simulink model "gm_sampleModel1484_2_sub"  (R2023a)
settings: Solver=VariableStepAuto  StartTime=0.0  StopTime=10.0  RelTol=1e-3
libraries: hdlsllib x2, simulink x2
settings Model: Creator=user1  LastModifiedBy=user1
settings OptimizationCC: BlockReduction=off  ConditionallyExecuteInputs=off
settings DebuggingCC: InheritedTsInSrcMsg=none

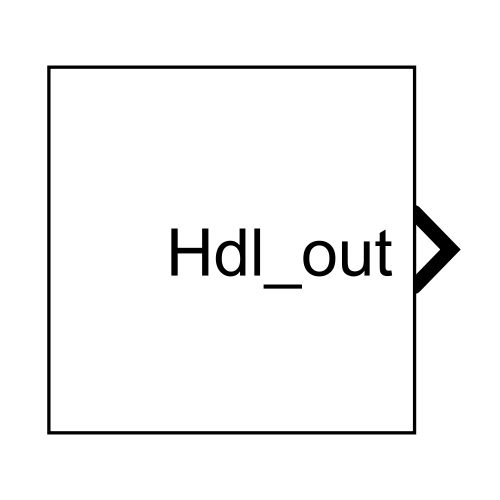
[thumbnail: Simulink's stored preview of the top-level diagram]
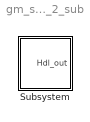
== system gm_sampleModel1484_2_sub ==
  Subsystem : Subsystem

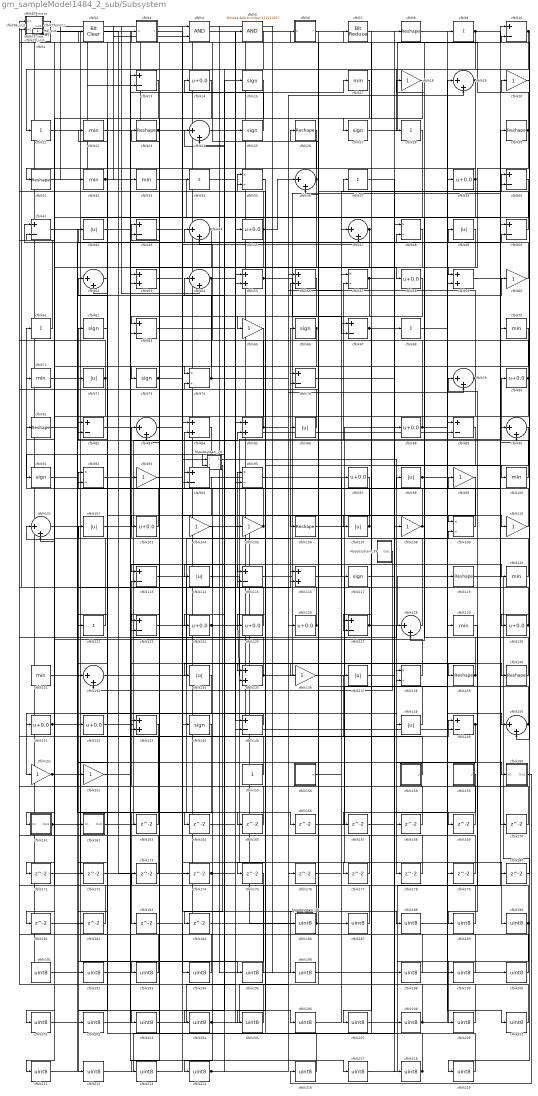
== system gm_sampleModel1484_2_sub/Subsystem ==
  Mysubsystem_20 : Subsystem
  Mysubsystem_38 : Subsystem
  Mysubsystem_39 : Subsystem
  cfblk1 : hdlsllib/Logic and Bit Operations/Bit Concat  numInputs=2
  cfblk{10,13,40..41,43,50,63,67,76,82,89,94,113,115,123,127,145,149} (18 alike) : Sum  Inputs=+-  OutDataTypeStr=uint8
  cfblk{17,22,32..33,70..71,100,120,129,131} (10 alike) : MinMax  OutDataTypeStr=uint8
  cfblk{19,24,36,44,47,52,54,79,83,90,101,128,132,150} (14 alike) : Sum  Inputs=|++  OutDataTypeStr=uint8
  cfblk{42,49,72,86,98,102,107,114,134,137,148} (11 alike) : Abs  OutDataTypeStr=uint8  SaturateOnIntegerOverflow=off
  cfblk{14,39,45,58,80,88,97,103,124..126,130,141..142} (14 alike) : Bias  Bias=0.0  SaturateOnIntegerOverflow=off
  cfblk{18,20,60,65,93,99,104..105,108,110,136,151..152} (13 alike) : Gain  OutDataTypeStr=uint8
  cfblk{8,23,26,30..31,81,106,119,139..140} (10 alike) : Reshape
  cfblk{35,48,57,74,92,95,109,138} (8 alike) : Product  Inputs=*/  OutDataTypeStr=uint8  RndMeth=Zero  SaturateOnIntegerOverflow=on
  cfblk112_inst : Subsystem
  cfblk{53,55..56,59,84..85,116,135,143} (9 alike) : Sum  OutDataTypeStr=uint8
  cfblk{15,25,27,62,66,73,91,117,144} (9 alike) : Signum
  cfblk11_inst : Subsystem
  cfblk121_inst : Subsystem
  cfblk{9,21,28,34,37,61,68,122} (8 alike) : Sum  Inputs=+  OutDataTypeStr=uint8
  cfblk12_inst : Subsystem
  cfblk146_inst : Subsystem
  cfblk147_inst : Subsystem
  cfblk155 : Constant  OutDataTypeStr=uint8  SampleTime=-1
  cfblk156 : Subsystem  mask(Counter Free-Running){NumBits=double(16), tsamp=double(-1)}
      mask prompts: NumBits "Simulink:masks:NumberOfBits_MP"; tsamp "Simulink:masks:SampleTime_MP"
      mask help: Simulink:masks:CounterFreeRunning_MD
  cfblk158 : Subsystem  mask(Counter Limited){uplimit=double(7), tsamp=double(-1)}
      mask prompts: uplimit "Simulink:masks:UpperLimit_MP"; tsamp "Simulink:masks:SampleTime_MP"
      mask help: Simulink:masks:CounterLimited_MD
      mask init:
      | nbits = double(8);
      | tsamp = double(-1);
      | uplimit = double(7);
  cfblk159 : Subsystem  mask(Counter Free-Running){NumBits=double(16), tsamp=double(-1)}
      mask prompts: NumBits "Simulink:masks:NumberOfBits_MP"; tsamp "Simulink:masks:SampleTime_MP"
      mask help: Simulink:masks:CounterFreeRunning_MD
  cfblk160 : Subsystem
  cfblk161 : Subsystem
  cfblk162 : Subsystem
  cfblk{163..184} (22 alike) : Delay  SampleTime=1
  cfblk16_inst : Subsystem
  cfblk{186..196,198..214,216..219} (32 alike) : DataTypeConversion  OutDataTypeStr=uint8  SaturateOnIntegerOverflow=off  RndMeth=Floor
  cfblk2 : simulink/Logic and Bit Operations/Bit Clear  iBit=0
      settings: LibrarySourceBlock=|
      | hdlsllib/Logic and Bit
      | Operations/Bit Clear
  cfblk29_inst : Subsystem
  cfblk3 : Subsystem  mask(Detect Fall Nonpositive){vinit=double(0), InputProcessing=Elements as channels (sample based), OutDataTypeStr=uint8}
      mask prompts: vinit "Simulink:masks:InitialCondition_MP"; InputProcessing "Simulink:masks:InputProcessing_MP"; OutDataTypeStr "Simulink:masks:OutputDataType_MP"
      mask help: Simulink:masks:DetectFallNonpositive_MD
      mask init:
      | InputProcessing = 'Elements as channels (sample based)';
      | OutDataTypeStr = 'uint8';
      | vinit = double(0);
      mask TypeOptions InputProcessing: Simulink:masks:ColumnsAsChannelsFrameBased | Simulink:masks:ElementsAsChannelsSampleBased
      mask TypeOptions OutDataTypeStr: Simulink:masks:uint8 | Simulink:masks:boolean
      mask Display: fprintf('U <= 0\n&  NOT\nU/z <= 0')
  cfblk4 : Logic  AllPortsSameDT=off  OutDataTypeStr=boolean
  cfblk5 : simulink/Logic and Bit Operations/Bitwise Operator  logicop=AND  UseBitMask=on  BitMask=bin2dec('11011001')  BitMaskRealWorld=Stored Integer
      settings: LibrarySourceBlock=|
      | hdlsllib/Logic and Bit
      | Operations/Bitwise
      | Operator
  cfblk6 : Subsystem  mask(Detect Rise Positive){vinit=double(0), InputProcessing=Elements as channels (sample based), OutDataTypeStr=uint8}
      mask prompts: vinit "Simulink:masks:InitialCondition_MP"; InputProcessing "Simulink:masks:InputProcessing_MP"; OutDataTypeStr "Simulink:masks:OutputDataType_MP"
      mask help: Simulink:masks:DetectRisePositive_MD
      mask init:
      | InputProcessing = 'Elements as channels (sample based)';
      | OutDataTypeStr = 'uint8';
      | vinit = double(0);
      mask TypeOptions InputProcessing: Simulink:masks:ColumnsAsChannelsFrameBased | Simulink:masks:ElementsAsChannelsSampleBased
      mask TypeOptions OutDataTypeStr: Simulink:masks:uint8 | Simulink:masks:boolean
      mask Display: fprintf('U > 0\n&  NOT\nU/z > 0')
  cfblk7 : hdlsllib/Logic and Bit Operations/Bit Reduce  mode=AND
  cfblk75_inst : Subsystem
  cfblk77_inst : Subsystem
  cfblk87_inst : Subsystem
  cfblk96_inst : Subsystem
  Hdl_out : Outport  OutDataTypeStr=uint8  SampleTime=1
  wires:
  Mysubsystem_20/1(Out1) -> cfblk178/1
  Mysubsystem_20/2(Out2) -> cfblk184/1
  Mysubsystem_38/1(Out1) -> cfblk104/1
  Mysubsystem_39/1(Out1) -> cfblk132/2
  cfblk1/1 -> cfblk193/1
  cfblk10/1 -> cfblk150/2, cfblk21/1
  cfblk100/1 -> cfblk62/1
  cfblk101/1 -> cfblk206/1
  cfblk102/1 -> cfblk85/2
  cfblk103/1 -> cfblk92/1
  cfblk104/1 -> cfblk214/1
  cfblk105/1 -> cfblk84/2, cfblk83/1
  cfblk106/1 -> cfblk88/1
  cfblk107/1 -> cfblk43/1, cfblk74/2
  cfblk108/1 -> cfblk24/2, cfblk24/1
  cfblk109/1 -> cfblk85/1
  cfblk11_inst/1(out1) -> cfblk9/1
  cfblk110/1 -> cfblk61/1
  cfblk112_inst/1(out1) -> cfblk54/2
  cfblk113/1 -> cfblk139/1
  cfblk114/1 -> cfblk177/1
  cfblk115/1 -> cfblk50/2
  cfblk116/1 -> cfblk190/1
  cfblk117/1 -> cfblk8/1
  cfblk119/1 -> cfblk219/1
  cfblk12_inst/1(out1) -> cfblk97/1
  cfblk120/1 -> cfblk93/1
  cfblk121_inst/1(out1) -> cfblk4/2, cfblk131/1
  cfblk122/1 -> cfblk81/1
  cfblk123/1 -> cfblk166/1
  cfblk124/1 -> cfblk135/2, cfblk57/2, cfblk138/2
  cfblk125/1 -> cfblk95/1
  cfblk126/1 -> cfblk75_inst/2(in2), cfblk11_inst/2(in2), cfblk35/1
  cfblk127/1 -> cfblk41/2, cfblk119/1
  cfblk128/1 -> cfblk112_inst/1(in1)
  cfblk129/1 -> cfblk189/1
  cfblk13/1 -> cfblk142/1
  cfblk130/1 -> cfblk94/1, cfblk66/1, cfblk52/2
  cfblk131/1 -> cfblk148/1
  cfblk132/1 -> cfblk86/1
  cfblk134/1 -> cfblk151/1
  cfblk135/1 -> cfblk80/1, cfblk16_inst/2(in2)
  cfblk136/1 -> cfblk50/1
  cfblk137/1 -> cfblk169/1
  cfblk138/1 -> cfblk71/1
  cfblk139/1 -> cfblk29_inst/1(in1), cfblk134/1
  cfblk14/1 -> cfblk174/1
  cfblk140/1 -> cfblk42/1
  cfblk141/1 -> cfblk82/1, cfblk165/1
  cfblk142/1 -> cfblk55/1
  cfblk143/1 -> cfblk212/1
  cfblk144/1 -> cfblk183/1
  cfblk145/1 -> cfblk141/1
  cfblk146_inst/1(out1) -> cfblk25/1
  cfblk147_inst/1(out1) -> cfblk200/1
  cfblk148/1 -> cfblk7/1
  cfblk149/1 -> cfblk99/1, cfblk168/1
  cfblk15/1 -> cfblk73/1
  cfblk150/1 -> cfblk26/1, cfblk20/1
  cfblk151/1 -> cfblk94/2, cfblk129/1
  cfblk152/1 -> cfblk13/1
  cfblk155/1 -> cfblk54/1
  cfblk156/1(y) -> cfblk47/1
  cfblk158/1(y) -> cfblk82/2
  cfblk159/1(y) -> cfblk207/1
  cfblk16_inst/1(out1) -> cfblk33/1
  cfblk160/1(Out1) -> cfblk216/1
  cfblk161/1(Out1) -> cfblk149/1, cfblk137/1
  cfblk162/1(Out1) -> cfblk128/1
  cfblk163/1 -> cfblk29_inst/2(in2)
  cfblk164/1 -> cfblk145/2
  cfblk165/1 -> cfblk113/2
  cfblk166/1 -> cfblk89/1
  cfblk167/1 -> cfblk109/2
  cfblk168/1 -> cfblk112_inst/2(in2)
  cfblk169/1 -> cfblk101/1
  cfblk17/1 -> cfblk201/1
  cfblk170/1 -> cfblk52/1
  cfblk171/1 -> cfblk95/2
  cfblk172/1 -> cfblk53/2
  cfblk173/1 -> cfblk147_inst/1(in1)
  cfblk174/1 -> cfblk55/2, Hdl_out/1
  cfblk175/1 -> cfblk192/1
  cfblk176/1 -> cfblk67/1
  cfblk177/1 -> cfblk77_inst/1(in1)
  cfblk178/1 -> cfblk44/1
  cfblk179/1 -> cfblk121_inst/2(in2)
  cfblk18/1 -> cfblk152/1
  cfblk180/1 -> cfblk10/2
  cfblk181/1 -> cfblk195/1
  cfblk182/1 -> cfblk87_inst/1(in1)
  cfblk183/1 -> cfblk194/1
  cfblk184/1 -> cfblk196/1
  cfblk186/1 -> cfblk53/1, cfblk102/1
  cfblk187/1 -> cfblk6/1(U)
  cfblk188/1 -> cfblk39/1
  cfblk189/1 -> cfblk3/1(U)
  cfblk19/1 -> cfblk203/1, cfblk202/1
  cfblk190/1 -> cfblk79/1, cfblk75_inst/1(in1), cfblk209/1
  cfblk191/1 -> cfblk116/1
  cfblk192/1 -> cfblk116/2
  cfblk193/1 -> cfblk147_inst/2(in2)
  cfblk194/1 -> cfblk1/1
  cfblk195/1 -> cfblk1/2
  cfblk196/1 -> cfblk199/1
  cfblk198/1 -> cfblk77_inst/2(in2)
  cfblk199/1 -> cfblk96_inst/1(in1)
  cfblk2/1 -> cfblk217/1
  cfblk20/1 -> cfblk130/1
  cfblk200/1 -> cfblk96_inst/2(in2)
  cfblk201/1 -> cfblk49/1
  cfblk202/1 -> cfblk17/1
  cfblk203/1 -> cfblk5/1
  cfblk204/1 -> cfblk45/1, cfblk176/1
  cfblk205/1 -> cfblk121_inst/1(in1)
  cfblk206/1 -> cfblk40/1
  cfblk207/1 -> cfblk40/2
  cfblk208/1 -> cfblk179/1, Mysubsystem_20/2(In2)
  cfblk209/1 -> cfblk76/1
  cfblk21/1 -> cfblk108/1
  cfblk210/1 -> cfblk76/2
  cfblk211/1 -> cfblk72/1
  cfblk212/1 -> cfblk48/1
  cfblk213/1 -> cfblk48/2
  cfblk214/1 -> cfblk79/2, cfblk15/1, cfblk126/1
  cfblk216/1 -> cfblk2/1
  cfblk217/1 -> cfblk70/1
  cfblk218/1 -> cfblk115/2, cfblk173/1
  cfblk219/1 -> cfblk37/1
  cfblk22/1 -> cfblk143/1
  cfblk23/1 -> cfblk144/1, cfblk115/1
  cfblk24/1 -> cfblk109/1
  cfblk25/1 -> cfblk14/1
  cfblk26/1 -> cfblk182/1
  cfblk27/1 -> cfblk10/1
  cfblk28/1 -> cfblk171/1
  cfblk29_inst/1(out1) -> cfblk187/1, cfblk13/2
  cfblk3/1(Y) -> cfblk188/1
  cfblk30/1 -> cfblk59/1, cfblk16_inst/1(in1)
  cfblk31/1 -> Mysubsystem_20/1(In1)
  cfblk32/1 -> cfblk43/2, cfblk140/1
  cfblk33/1 -> cfblk90/1
  cfblk34/1 -> cfblk145/1
  cfblk35/1 -> cfblk125/1
  cfblk36/1 -> cfblk63/1, cfblk146_inst/1(in1)
  cfblk37/1 -> cfblk218/1
  cfblk39/1 -> cfblk31/1, cfblk128/2
  cfblk4/1 -> cfblk105/1
  cfblk40/1 -> cfblk205/1
  cfblk41/1 -> cfblk164/1
  cfblk42/1 -> cfblk58/1
  cfblk43/1 -> cfblk136/1
  cfblk44/1 -> cfblk101/2, cfblk163/1
  cfblk45/1 -> cfblk63/2, cfblk36/1, cfblk12_inst/2(in2), cfblk175/1
  cfblk47/1 -> cfblk124/1, cfblk123/1
  cfblk48/1 -> cfblk211/1
  cfblk49/1 -> cfblk114/1
  cfblk5/1 -> cfblk204/1
  cfblk50/1 -> cfblk146_inst/2(in2)
  cfblk52/1 -> cfblk22/1
  cfblk53/1 -> cfblk106/1
  cfblk54/1 -> cfblk83/2, cfblk143/2, cfblk138/1
  cfblk55/1 -> cfblk67/2, cfblk30/1
  cfblk56/1 -> cfblk65/1
  cfblk57/1 -> cfblk213/1, cfblk100/1
  cfblk58/1 -> cfblk113/1
  cfblk59/1 -> cfblk90/2
  cfblk6/1(Y) -> cfblk186/1
  cfblk60/1 -> cfblk41/1
  cfblk61/1 -> cfblk12_inst/1(in1)
  cfblk62/1 -> cfblk162/1(In1)
  cfblk63/1 -> cfblk110/1
  cfblk65/1 -> cfblk122/1
  cfblk66/1 -> cfblk74/1, cfblk181/1
  cfblk67/1 -> cfblk127/2, cfblk68/1
  cfblk68/1 -> cfblk19/1
  cfblk7/1 -> cfblk27/1
  cfblk70/1 -> cfblk132/1
  cfblk71/1 -> cfblk160/1(In1)
  cfblk72/1 -> cfblk11_inst/1(in1), cfblk92/2
  cfblk73/1 -> cfblk84/1, cfblk47/2
  cfblk74/1 -> cfblk4/1, cfblk19/2
  cfblk75_inst/1(out1) -> cfblk89/2, cfblk34/1
  cfblk76/1 -> cfblk208/1
  cfblk77_inst/1(out1) -> cfblk32/1
  cfblk79/1 -> cfblk36/2, cfblk107/1
  cfblk8/1 -> cfblk150/1
  cfblk80/1 -> cfblk123/2, cfblk35/2, cfblk161/1(In1)
  cfblk81/1 -> cfblk60/1
  cfblk82/1 -> cfblk120/1
  cfblk83/1 -> cfblk180/1
  cfblk84/1 -> cfblk91/1
  cfblk85/1 -> cfblk23/1, cfblk57/1
  cfblk86/1 -> cfblk87_inst/2(in2)
  cfblk87_inst/1(out1) -> cfblk191/1, cfblk149/2
  cfblk88/1 -> cfblk59/2, cfblk44/2
  cfblk89/1 -> cfblk135/1
  cfblk9/1 -> cfblk170/1, cfblk28/1
  cfblk90/1 -> cfblk127/1
  cfblk91/1 -> cfblk98/1
  cfblk92/1 -> cfblk56/2
  cfblk93/1 -> cfblk56/1
  cfblk94/1 -> cfblk172/1
  cfblk95/1 -> cfblk117/1
  cfblk96_inst/1(out1) -> cfblk198/1
  cfblk97/1 -> cfblk103/1
  cfblk98/1 -> cfblk210/1, cfblk18/1
  cfblk99/1 -> cfblk167/1

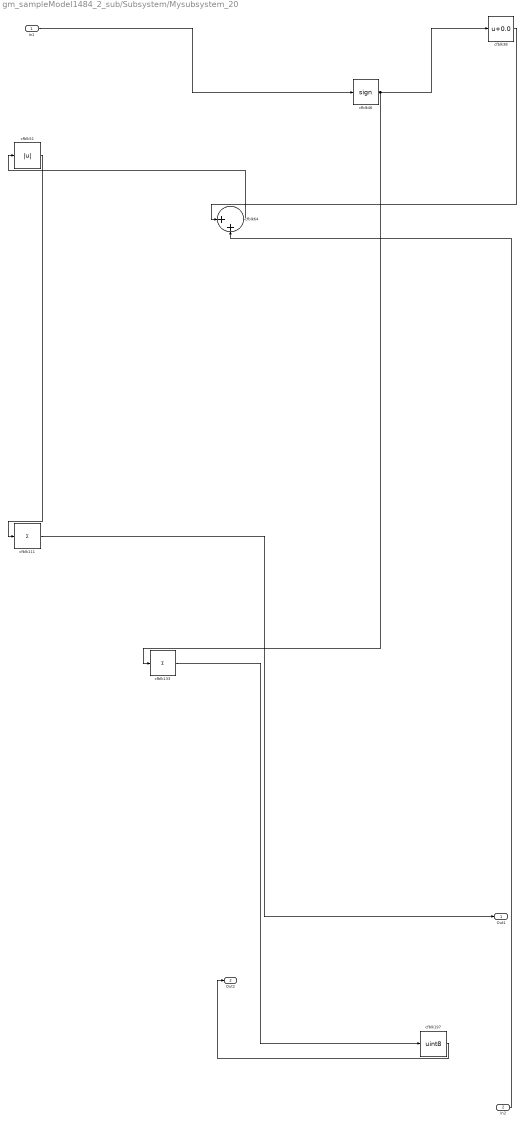
== system gm_sampleModel1484_2_sub/Subsystem/Mysubsystem_20 ==
  In1 : Inport  OutDataTypeStr=uint8  PortDimensions=1  SampleTime=1
  In2 : Inport  Port=2  OutDataTypeStr=uint8  PortDimensions=1  SampleTime=1
  cfblk111 : Sum  Inputs=+
  cfblk133 : Sum  Inputs=+
  cfblk197 : DataTypeConversion  OutDataTypeStr=uint8  SaturateOnIntegerOverflow=off  RndMeth=Floor
  cfblk38 : Bias  Bias=0.0  SaturateOnIntegerOverflow=off
  cfblk46 : Signum
  cfblk51 : Abs  SaturateOnIntegerOverflow=off
  cfblk64 : Sum  Inputs=|++
  Out1 : Outport  SampleTime=1
  Out2 : Outport  Port=2  SampleTime=1
  wires:
  In1/1 -> cfblk46/1
  In2/1 -> cfblk64/2
  cfblk111/1 -> Out1/1
  cfblk133/1 -> cfblk197/1
  cfblk197/1 -> Out2/1
  cfblk38/1 -> cfblk64/1
  cfblk46/1 -> cfblk38/1, cfblk133/1
  cfblk51/1 -> cfblk111/1
  cfblk64/1 -> cfblk51/1

== system gm_sampleModel1484_2_sub/Subsystem/Mysubsystem_38 ==
  cfblk157 : Subsystem  mask(Counter Free-Running){NumBits=double(16), tsamp=double(-1)}
      mask prompts: NumBits "Simulink:masks:NumberOfBits_MP"; tsamp "Simulink:masks:SampleTime_MP"
      mask help: Simulink:masks:CounterFreeRunning_MD
  cfblk215 : DataTypeConversion  OutDataTypeStr=uint8  SaturateOnIntegerOverflow=off  RndMeth=Floor
  Out1 : Outport  SampleTime=1
  wires:
  cfblk157/1(y) -> cfblk215/1
  cfblk215/1 -> Out1/1

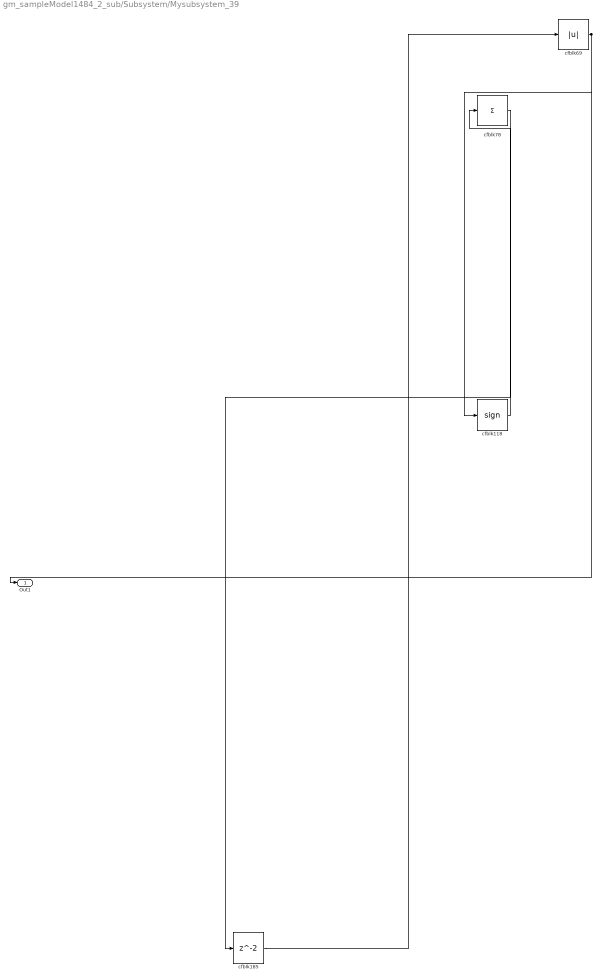
== system gm_sampleModel1484_2_sub/Subsystem/Mysubsystem_39 ==
  cfblk118 : Signum
  cfblk185 : Delay  SampleTime=1
  cfblk69 : Abs  SaturateOnIntegerOverflow=off
  cfblk78 : Sum  Inputs=+
  Out1 : Outport  SampleTime=1
  wires:
  cfblk118/1 -> cfblk78/1
  cfblk185/1 -> cfblk69/1
  cfblk69/1 -> cfblk118/1, Out1/1
  cfblk78/1 -> cfblk185/1

== system gm_sampleModel1484_2_sub/Subsystem/cfblk112_inst ==
  in1 : Inport  OutDataTypeStr=uint8  SampleTime=1
  in2 : Inport  Port=2  OutDataTypeStr=uint8  SampleTime=1
  mul_cfblk112_dotp_mulcomp : Product  Inputs=**  OutDataTypeStr=uint8  SampleTime=1
  out1 : Outport  OutDataTypeStr=uint8  SampleTime=1
  wires:
  in1/1 -> mul_cfblk112_dotp_mulcomp/1
  in2/1 -> mul_cfblk112_dotp_mulcomp/2
  mul_cfblk112_dotp_mulcomp/1 -> out1/1

== system gm_sampleModel1484_2_sub/Subsystem/cfblk11_inst ==
  in1 : Inport  OutDataTypeStr=uint8  SampleTime=1
  in2 : Inport  Port=2  OutDataTypeStr=uint8  SampleTime=1
  mul_cfblk11_dotp_mulcomp : Product  Inputs=**  OutDataTypeStr=uint8  SampleTime=1
  out1 : Outport  OutDataTypeStr=uint8  SampleTime=1
  wires:
  in1/1 -> mul_cfblk11_dotp_mulcomp/1
  in2/1 -> mul_cfblk11_dotp_mulcomp/2
  mul_cfblk11_dotp_mulcomp/1 -> out1/1

== system gm_sampleModel1484_2_sub/Subsystem/cfblk121_inst ==
  in1 : Inport  OutDataTypeStr=uint8  SampleTime=1
  in2 : Inport  Port=2  OutDataTypeStr=uint8  SampleTime=1
  mul_cfblk121_dotp_mulcomp : Product  Inputs=**  OutDataTypeStr=uint8  SampleTime=1
  out1 : Outport  OutDataTypeStr=uint8  SampleTime=1
  wires:
  in1/1 -> mul_cfblk121_dotp_mulcomp/1
  in2/1 -> mul_cfblk121_dotp_mulcomp/2
  mul_cfblk121_dotp_mulcomp/1 -> out1/1

== system gm_sampleModel1484_2_sub/Subsystem/cfblk12_inst ==
  in1 : Inport  OutDataTypeStr=uint8  SampleTime=1
  in2 : Inport  Port=2  OutDataTypeStr=uint8  SampleTime=1
  mul_cfblk12_dotp_mulcomp : Product  Inputs=**  OutDataTypeStr=uint8  SampleTime=1
  out1 : Outport  OutDataTypeStr=uint8  SampleTime=1
  wires:
  in1/1 -> mul_cfblk12_dotp_mulcomp/1
  in2/1 -> mul_cfblk12_dotp_mulcomp/2
  mul_cfblk12_dotp_mulcomp/1 -> out1/1

== system gm_sampleModel1484_2_sub/Subsystem/cfblk146_inst ==
  in1 : Inport  OutDataTypeStr=uint8  SampleTime=1
  in2 : Inport  Port=2  OutDataTypeStr=uint8  SampleTime=1
  mul_cfblk146_dotp_mulcomp : Product  Inputs=**  OutDataTypeStr=uint8  SampleTime=1
  out1 : Outport  OutDataTypeStr=uint8  SampleTime=1
  wires:
  in1/1 -> mul_cfblk146_dotp_mulcomp/1
  in2/1 -> mul_cfblk146_dotp_mulcomp/2
  mul_cfblk146_dotp_mulcomp/1 -> out1/1

== system gm_sampleModel1484_2_sub/Subsystem/cfblk147_inst ==
  in1 : Inport  OutDataTypeStr=uint8  SampleTime=1
  in2 : Inport  Port=2  OutDataTypeStr=uint8  SampleTime=1
  mul_cfblk147_dotp_mulcomp : Product  Inputs=**  OutDataTypeStr=uint8  SampleTime=1
  out1 : Outport  OutDataTypeStr=uint8  SampleTime=1
  wires:
  in1/1 -> mul_cfblk147_dotp_mulcomp/1
  in2/1 -> mul_cfblk147_dotp_mulcomp/2
  mul_cfblk147_dotp_mulcomp/1 -> out1/1

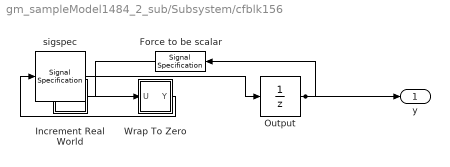
== system gm_sampleModel1484_2_sub/Subsystem/cfblk156 ==
  Force to be scalar : SignalSpecification  DisableCoverage=on  Dimensions=1
  Increment Real World : Subsystem  mask(Real World Value Increment){}
      mask help: Simulink:masks:RealWorldValueIncrement_MD
      mask Display: disp('V++')
  Output : UnitDelay  InitialCondition=0.0  SampleTime=tsamp  HasFrameUpgradeWarning=on
  Wrap To Zero : Subsystem  mask(Wrap To Zero){Threshold=double(65535)}
      mask prompts: Threshold "Simulink:masks:Threshold_MP"
      mask help: Simulink:masks:WrapToZero_MD
  sigspec : SignalSpecification  OutDataTypeStr=uint16  Dimensions=1
  y : Outport  SampleTime=1
  wires:
  Force to be scalar/1 -> Increment Real World/1(u)
  Increment Real World/1(y) -> Wrap To Zero/1(U)
  Output/1 -> Force to be scalar/1, y/1
  Wrap To Zero/1(Y) -> sigspec/1
  sigspec/1 -> Output/1

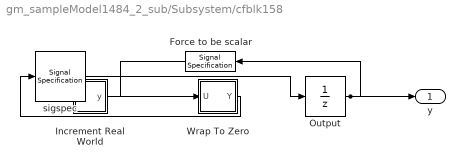
== system gm_sampleModel1484_2_sub/Subsystem/cfblk158 ==
  Force to be scalar : SignalSpecification  DisableCoverage=on  Dimensions=1
  Increment Real World : Subsystem  mask(Real World Value Increment){}
      mask help: Simulink:masks:RealWorldValueIncrement_MD
      mask Display: disp('V++')
  Output : UnitDelay  InitialCondition=0.0  SampleTime=tsamp  HasFrameUpgradeWarning=on
  Wrap To Zero : Subsystem  mask(Wrap To Zero){Threshold=double(7)}
      mask prompts: Threshold "Simulink:masks:Threshold_MP"
      mask help: Simulink:masks:WrapToZero_MD
  sigspec : SignalSpecification  OutDataTypeStr=uint8  Dimensions=1
  y : Outport  SampleTime=1
  wires:
  Force to be scalar/1 -> Increment Real World/1(u)
  Increment Real World/1(y) -> Wrap To Zero/1(U)
  Output/1 -> Force to be scalar/1, y/1
  Wrap To Zero/1(Y) -> sigspec/1
  sigspec/1 -> Output/1

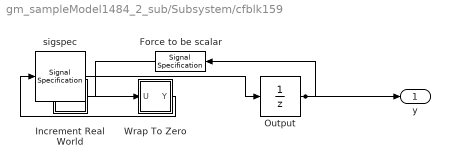
== system gm_sampleModel1484_2_sub/Subsystem/cfblk159 ==
  Force to be scalar : SignalSpecification  DisableCoverage=on  Dimensions=1
  Increment Real World : Subsystem  mask(Real World Value Increment){}
      mask help: Simulink:masks:RealWorldValueIncrement_MD
      mask Display: disp('V++')
  Output : UnitDelay  InitialCondition=0.0  SampleTime=tsamp  HasFrameUpgradeWarning=on
  Wrap To Zero : Subsystem  mask(Wrap To Zero){Threshold=double(65535)}
      mask prompts: Threshold "Simulink:masks:Threshold_MP"
      mask help: Simulink:masks:WrapToZero_MD
  sigspec : SignalSpecification  OutDataTypeStr=uint16  Dimensions=1
  y : Outport  SampleTime=1
  wires:
  Force to be scalar/1 -> Increment Real World/1(u)
  Increment Real World/1(y) -> Wrap To Zero/1(U)
  Output/1 -> Force to be scalar/1, y/1
  Wrap To Zero/1(Y) -> sigspec/1
  sigspec/1 -> Output/1

== system gm_sampleModel1484_2_sub/Subsystem/cfblk160 ==
  In1 : Inport  OutDataTypeStr=uint8  PortDimensions=1  SampleTime=1
  Out1 : Outport  SampleTime=1
  wires:
  In1/1 -> Out1/1

== system gm_sampleModel1484_2_sub/Subsystem/cfblk161 ==
  In1 : Inport  OutDataTypeStr=uint8  PortDimensions=1  SampleTime=1
  Out1 : Outport  SampleTime=1
  wires:
  In1/1 -> Out1/1

== system gm_sampleModel1484_2_sub/Subsystem/cfblk162 ==
  In1 : Inport  OutDataTypeStr=uint8  PortDimensions=1  SampleTime=1
  Out1 : Outport  SampleTime=1
  wires:
  In1/1 -> Out1/1

== system gm_sampleModel1484_2_sub/Subsystem/cfblk16_inst ==
  in1 : Inport  OutDataTypeStr=uint8  SampleTime=1
  in2 : Inport  Port=2  OutDataTypeStr=uint8  SampleTime=1
  mul_cfblk16_dotp_mulcomp : Product  Inputs=**  OutDataTypeStr=uint8  SampleTime=1
  out1 : Outport  OutDataTypeStr=uint8  SampleTime=1
  wires:
  in1/1 -> mul_cfblk16_dotp_mulcomp/1
  in2/1 -> mul_cfblk16_dotp_mulcomp/2
  mul_cfblk16_dotp_mulcomp/1 -> out1/1

== system gm_sampleModel1484_2_sub/Subsystem/cfblk29_inst ==
  in1 : Inport  OutDataTypeStr=uint8  SampleTime=1
  in2 : Inport  Port=2  OutDataTypeStr=uint8  SampleTime=1
  mul_cfblk29_dotp_mulcomp : Product  Inputs=**  OutDataTypeStr=uint8  SampleTime=1
  out1 : Outport  OutDataTypeStr=uint8  SampleTime=1
  wires:
  in1/1 -> mul_cfblk29_dotp_mulcomp/1
  in2/1 -> mul_cfblk29_dotp_mulcomp/2
  mul_cfblk29_dotp_mulcomp/1 -> out1/1

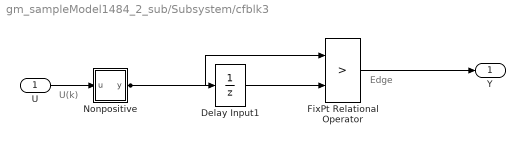
== system gm_sampleModel1484_2_sub/Subsystem/cfblk3 ==
  note: U(k)
  note: Edge
  U : Inport  OutDataTypeStr=uint8  SampleTime=1
  Delay Input1 : UnitDelay  Description=Store in Global RAM  DisableCoverage=on  InitialCondition=vinit  SampleTime=-1  HasFrameUpgradeWarning=on
  FixPt Relational Operator : RelationalOperator  Operator=>  OutDataTypeStr=fixdt(0, 8)  ZeroCross=off  InputSameDT=off
  Nonpositive : Subsystem  mask(Compare To Zero){relop=<=, OutDataTypeStr=boolean, ZeroCross=off}
      mask prompts: relop "Simulink:masks:Operator_MP"; OutDataTypeStr "Simulink:masks:OutputDataType_MP"; ZeroCross "Simulink:masks:EnableZerocrossingDetection_MP"
      mask help: Simulink:masks:CompareToZero_MD
      mask init:
      | OutDataTypeStr = 'boolean';
      | ZeroCross = 'off';
      | blkName = 'sampleModel1484_2_sub/Subsystem/cfblk3/Nonpositive';
      | relop = '<=';
      | setValue = 'boolean';
      mask TypeOptions relop: == | ~= | < | <= | >= | >
      mask TypeOptions OutDataTypeStr: Simulink:masks:uint8 | Simulink:masks:boolean
      mask Callback ZeroCross: sl('zeroCrossEnable', gcbh);
      mask Display: disp([relop,' 0'])
  Y : Outport  SampleTime=1
  wires:
  U/1 -> Nonpositive/1(u)
  Delay Input1/1 -> FixPt Relational Operator/2
  FixPt Relational Operator/1 -> Y/1
  Nonpositive/1(y) -> FixPt Relational Operator/1, Delay Input1/1

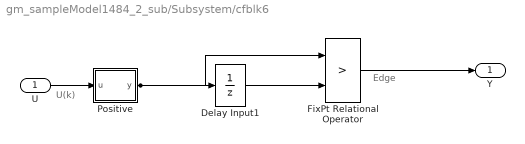
== system gm_sampleModel1484_2_sub/Subsystem/cfblk6 ==
  note: U(k)
  note: Edge
  U : Inport  OutDataTypeStr=uint8  SampleTime=1
  Delay Input1 : UnitDelay  Description=Store in Global RAM  DisableCoverage=on  InitialCondition=vinit  SampleTime=-1  HasFrameUpgradeWarning=on
  FixPt Relational Operator : RelationalOperator  Operator=>  OutDataTypeStr=fixdt(0, 8)  ZeroCross=off  InputSameDT=off
  Positive : Subsystem  mask(Compare To Zero){relop=>, OutDataTypeStr=boolean, ZeroCross=off}
      mask prompts: relop "Simulink:masks:Operator_MP"; OutDataTypeStr "Simulink:masks:OutputDataType_MP"; ZeroCross "Simulink:masks:EnableZerocrossingDetection_MP"
      mask help: Simulink:masks:CompareToZero_MD
      mask init:
      | OutDataTypeStr = 'boolean';
      | ZeroCross = 'off';
      | blkName = 'sampleModel1484_2_sub/Subsystem/cfblk6/Positive';
      | relop = '>';
      | setValue = 'boolean';
      mask TypeOptions relop: == | ~= | < | <= | >= | >
      mask TypeOptions OutDataTypeStr: Simulink:masks:uint8 | Simulink:masks:boolean
      mask Callback ZeroCross: sl('zeroCrossEnable', gcbh);
      mask Display: disp([relop,' 0'])
  Y : Outport  SampleTime=1
  wires:
  U/1 -> Positive/1(u)
  Delay Input1/1 -> FixPt Relational Operator/2
  FixPt Relational Operator/1 -> Y/1
  Positive/1(y) -> FixPt Relational Operator/1, Delay Input1/1

== system gm_sampleModel1484_2_sub/Subsystem/cfblk75_inst ==
  in1 : Inport  OutDataTypeStr=uint8  SampleTime=1
  in2 : Inport  Port=2  OutDataTypeStr=uint8  SampleTime=1
  mul_cfblk75_dotp_mulcomp : Product  Inputs=**  OutDataTypeStr=uint8  SampleTime=1
  out1 : Outport  OutDataTypeStr=uint8  SampleTime=1
  wires:
  in1/1 -> mul_cfblk75_dotp_mulcomp/1
  in2/1 -> mul_cfblk75_dotp_mulcomp/2
  mul_cfblk75_dotp_mulcomp/1 -> out1/1

== system gm_sampleModel1484_2_sub/Subsystem/cfblk77_inst ==
  in1 : Inport  OutDataTypeStr=uint8  SampleTime=1
  in2 : Inport  Port=2  OutDataTypeStr=uint8  SampleTime=1
  mul_cfblk77_dotp_mulcomp : Product  Inputs=**  OutDataTypeStr=uint8  SampleTime=1
  out1 : Outport  OutDataTypeStr=uint8  SampleTime=1
  wires:
  in1/1 -> mul_cfblk77_dotp_mulcomp/1
  in2/1 -> mul_cfblk77_dotp_mulcomp/2
  mul_cfblk77_dotp_mulcomp/1 -> out1/1

== system gm_sampleModel1484_2_sub/Subsystem/cfblk87_inst ==
  in1 : Inport  OutDataTypeStr=uint8  SampleTime=1
  in2 : Inport  Port=2  OutDataTypeStr=uint8  SampleTime=1
  mul_cfblk87_dotp_mulcomp : Product  Inputs=**  OutDataTypeStr=uint8  SampleTime=1
  out1 : Outport  OutDataTypeStr=uint8  SampleTime=1
  wires:
  in1/1 -> mul_cfblk87_dotp_mulcomp/1
  in2/1 -> mul_cfblk87_dotp_mulcomp/2
  mul_cfblk87_dotp_mulcomp/1 -> out1/1

== system gm_sampleModel1484_2_sub/Subsystem/cfblk96_inst ==
  in1 : Inport  OutDataTypeStr=uint8  SampleTime=1
  in2 : Inport  Port=2  OutDataTypeStr=uint8  SampleTime=1
  mul_cfblk96_dotp_mulcomp : Product  Inputs=**  OutDataTypeStr=uint8  SampleTime=1
  out1 : Outport  OutDataTypeStr=uint8  SampleTime=1
  wires:
  in1/1 -> mul_cfblk96_dotp_mulcomp/1
  in2/1 -> mul_cfblk96_dotp_mulcomp/2
  mul_cfblk96_dotp_mulcomp/1 -> out1/1

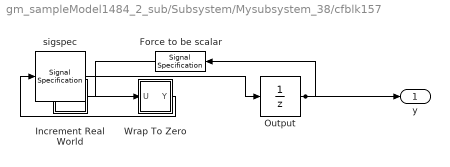
== system gm_sampleModel1484_2_sub/Subsystem/Mysubsystem_38/cfblk157 ==
  Force to be scalar : SignalSpecification  DisableCoverage=on  Dimensions=1
  Increment Real World : Subsystem  mask(Real World Value Increment){}
      mask help: Simulink:masks:RealWorldValueIncrement_MD
      mask Display: disp('V++')
  Output : UnitDelay  InitialCondition=0.0  SampleTime=tsamp  HasFrameUpgradeWarning=on
  Wrap To Zero : Subsystem  mask(Wrap To Zero){Threshold=double(65535)}
      mask prompts: Threshold "Simulink:masks:Threshold_MP"
      mask help: Simulink:masks:WrapToZero_MD
  sigspec : SignalSpecification  OutDataTypeStr=uint16  Dimensions=1
  y : Outport  SampleTime=1
  wires:
  Force to be scalar/1 -> Increment Real World/1(u)
  Increment Real World/1(y) -> Wrap To Zero/1(U)
  Output/1 -> Force to be scalar/1, y/1
  Wrap To Zero/1(Y) -> sigspec/1
  sigspec/1 -> Output/1

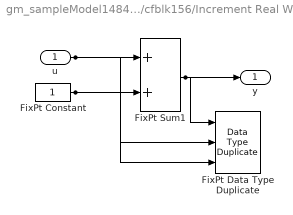
== system gm_sampleModel1484_2_sub/Subsystem/cfblk156/Increment Real World ==
  u : Inport  OutDataTypeStr=uint16  SampleTime=1
  FixPt Constant : Constant  DisableCoverage=on  OutDataTypeStr=Inherit: Inherit via back propagation  SampleTime=-1
  FixPt Data Type Duplicate : DataTypeDuplicate  DisableCoverage=on  NumInputPorts=3
  FixPt Sum1 : Sum  InputSameDT=on  OutDataTypeStr=Inherit: Inherit via back propagation  LockScale=on
  y : Outport  SampleTime=1
  wires:
  u/1 -> FixPt Sum1/1, FixPt Data Type Duplicate/2
  FixPt Constant/1 -> FixPt Sum1/2, FixPt Data Type Duplicate/3
  FixPt Sum1/1 -> FixPt Data Type Duplicate/1, y/1

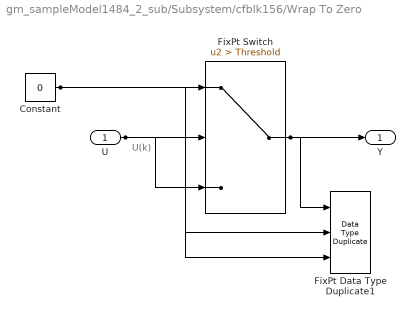
== system gm_sampleModel1484_2_sub/Subsystem/cfblk156/Wrap To Zero ==
  note: U(k)
  U : Inport  OutDataTypeStr=uint16  SampleTime=1
  Constant : Constant  DisableCoverage=on  Value=0  OutDataTypeStr=Inherit: Inherit via back propagation  SampleTime=-1
  FixPt Data Type Duplicate1 : DataTypeDuplicate  DisableCoverage=on  NumInputPorts=3
  FixPt Switch : Switch  Criteria=u2 > Threshold  Threshold=Threshold  OutDataTypeStr=Inherit: Inherit via back propagation  ZeroCross=off  SaturateOnIntegerOverflow=off  InputSameDT=off
  Y : Outport  SampleTime=1
  wires:
  U/1 -> FixPt Switch/3, FixPt Switch/2, FixPt Data Type Duplicate1/2
  Constant/1 -> FixPt Switch/1, FixPt Data Type Duplicate1/3
  FixPt Switch/1 -> FixPt Data Type Duplicate1/1, Y/1

== system gm_sampleModel1484_2_sub/Subsystem/cfblk158/Increment Real World ==
  u : Inport  OutDataTypeStr=uint8  SampleTime=1
  FixPt Constant : Constant  DisableCoverage=on  OutDataTypeStr=Inherit: Inherit via back propagation  SampleTime=-1
  FixPt Data Type Duplicate : DataTypeDuplicate  DisableCoverage=on  NumInputPorts=3
  FixPt Sum1 : Sum  InputSameDT=on  OutDataTypeStr=Inherit: Inherit via back propagation  LockScale=on
  y : Outport  SampleTime=1
  wires:
  u/1 -> FixPt Sum1/1, FixPt Data Type Duplicate/2
  FixPt Constant/1 -> FixPt Sum1/2, FixPt Data Type Duplicate/3
  FixPt Sum1/1 -> FixPt Data Type Duplicate/1, y/1

== system gm_sampleModel1484_2_sub/Subsystem/cfblk158/Wrap To Zero ==
  note: U(k)
  U : Inport  OutDataTypeStr=uint8  SampleTime=1
  Constant : Constant  DisableCoverage=on  Value=0  OutDataTypeStr=Inherit: Inherit via back propagation  SampleTime=-1
  FixPt Data Type Duplicate1 : DataTypeDuplicate  DisableCoverage=on  NumInputPorts=3
  FixPt Switch : Switch  Criteria=u2 > Threshold  Threshold=Threshold  OutDataTypeStr=Inherit: Inherit via back propagation  ZeroCross=off  SaturateOnIntegerOverflow=off  InputSameDT=off
  Y : Outport  SampleTime=1
  wires:
  U/1 -> FixPt Switch/3, FixPt Switch/2, FixPt Data Type Duplicate1/2
  Constant/1 -> FixPt Switch/1, FixPt Data Type Duplicate1/3
  FixPt Switch/1 -> FixPt Data Type Duplicate1/1, Y/1

== system gm_sampleModel1484_2_sub/Subsystem/cfblk159/Increment Real World ==
  u : Inport  OutDataTypeStr=uint16  SampleTime=1
  FixPt Constant : Constant  DisableCoverage=on  OutDataTypeStr=Inherit: Inherit via back propagation  SampleTime=-1
  FixPt Data Type Duplicate : DataTypeDuplicate  DisableCoverage=on  NumInputPorts=3
  FixPt Sum1 : Sum  InputSameDT=on  OutDataTypeStr=Inherit: Inherit via back propagation  LockScale=on
  y : Outport  SampleTime=1
  wires:
  u/1 -> FixPt Sum1/1, FixPt Data Type Duplicate/2
  FixPt Constant/1 -> FixPt Sum1/2, FixPt Data Type Duplicate/3
  FixPt Sum1/1 -> FixPt Data Type Duplicate/1, y/1

== system gm_sampleModel1484_2_sub/Subsystem/cfblk159/Wrap To Zero ==
  note: U(k)
  U : Inport  OutDataTypeStr=uint16  SampleTime=1
  Constant : Constant  DisableCoverage=on  Value=0  OutDataTypeStr=Inherit: Inherit via back propagation  SampleTime=-1
  FixPt Data Type Duplicate1 : DataTypeDuplicate  DisableCoverage=on  NumInputPorts=3
  FixPt Switch : Switch  Criteria=u2 > Threshold  Threshold=Threshold  OutDataTypeStr=Inherit: Inherit via back propagation  ZeroCross=off  SaturateOnIntegerOverflow=off  InputSameDT=off
  Y : Outport  SampleTime=1
  wires:
  U/1 -> FixPt Switch/3, FixPt Switch/2, FixPt Data Type Duplicate1/2
  Constant/1 -> FixPt Switch/1, FixPt Data Type Duplicate1/3
  FixPt Switch/1 -> FixPt Data Type Duplicate1/1, Y/1

== system gm_sampleModel1484_2_sub/Subsystem/cfblk3/Nonpositive ==
  u : Inport  OutDataTypeStr=uint8  SampleTime=1
  Compare : RelationalOperator  Operator=<=  OutDataTypeStr=boolean  ZeroCross=off
  Constant : Constant  DisableCoverage=on  Value=0  OutDataTypeStr=Inherit: Inherit via back propagation  SampleTime=-1  PreserveConstantTs=on
  y : Outport  SampleTime=1
  wires:
  u/1 -> Compare/1
  Compare/1 -> y/1
  Constant/1 -> Compare/2

== system gm_sampleModel1484_2_sub/Subsystem/cfblk6/Positive ==
  u : Inport  OutDataTypeStr=uint8  SampleTime=1
  Compare : RelationalOperator  Operator=>  OutDataTypeStr=boolean  ZeroCross=off
  Constant : Constant  DisableCoverage=on  Value=0  OutDataTypeStr=Inherit: Inherit via back propagation  SampleTime=-1  PreserveConstantTs=on
  y : Outport  SampleTime=1
  wires:
  u/1 -> Compare/1
  Compare/1 -> y/1
  Constant/1 -> Compare/2

== system gm_sampleModel1484_2_sub/Subsystem/Mysubsystem_38/cfblk157/Increment Real World ==
  u : Inport  OutDataTypeStr=uint16  SampleTime=1
  FixPt Constant : Constant  DisableCoverage=on  OutDataTypeStr=Inherit: Inherit via back propagation  SampleTime=-1
  FixPt Data Type Duplicate : DataTypeDuplicate  DisableCoverage=on  NumInputPorts=3
  FixPt Sum1 : Sum  InputSameDT=on  OutDataTypeStr=Inherit: Inherit via back propagation  LockScale=on
  y : Outport  SampleTime=1
  wires:
  u/1 -> FixPt Sum1/1, FixPt Data Type Duplicate/2
  FixPt Constant/1 -> FixPt Sum1/2, FixPt Data Type Duplicate/3
  FixPt Sum1/1 -> FixPt Data Type Duplicate/1, y/1

== system gm_sampleModel1484_2_sub/Subsystem/Mysubsystem_38/cfblk157/Wrap To Zero ==
  note: U(k)
  U : Inport  OutDataTypeStr=uint16  SampleTime=1
  Constant : Constant  DisableCoverage=on  Value=0  OutDataTypeStr=Inherit: Inherit via back propagation  SampleTime=-1
  FixPt Data Type Duplicate1 : DataTypeDuplicate  DisableCoverage=on  NumInputPorts=3
  FixPt Switch : Switch  Criteria=u2 > Threshold  Threshold=Threshold  OutDataTypeStr=Inherit: Inherit via back propagation  ZeroCross=off  SaturateOnIntegerOverflow=off  InputSameDT=off
  Y : Outport  SampleTime=1
  wires:
  U/1 -> FixPt Switch/3, FixPt Switch/2, FixPt Data Type Duplicate1/2
  Constant/1 -> FixPt Switch/1, FixPt Data Type Duplicate1/3
  FixPt Switch/1 -> FixPt Data Type Duplicate1/1, Y/1
